simulink model "lead_lag"  (R2015a)
settings: Solver=ode45  StartTime=0.0  StopTime=3999  RelTol=1e-3
undefined symbols (not defined in the file or in its folder): sigbuilder_block
libraries: powerlib_meascontrol x4
settings Model: CovSFcnEnable=off  Creator=MEHRDAD  LastModifiedBy=FaraDars
settings DebuggingCC: SolverPrmCheckMsg=warning

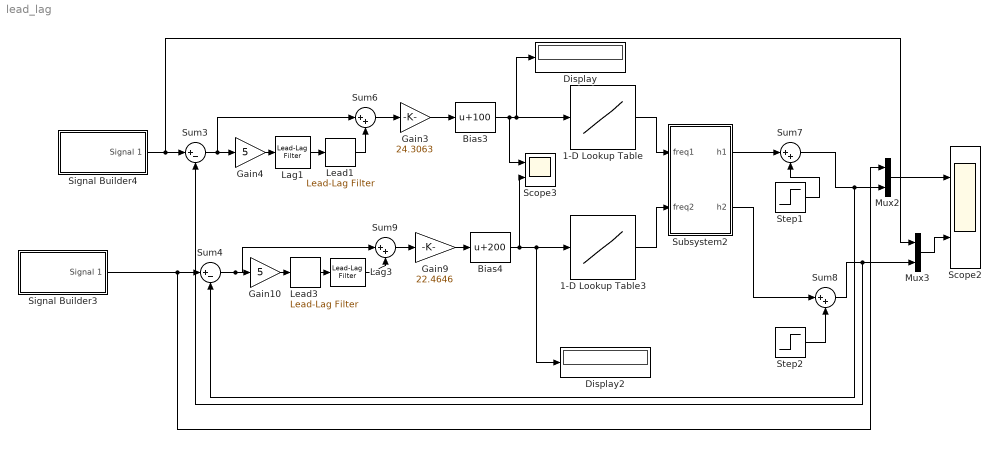
== system lead_lag ==
  1-D Lookup Table : Lookup_n-D  NumberOfTableDimensions=1  BreakpointsForDimension1="[163.87 211.67  227.76 244.4 261.62 274.69 289.41 301.46 318.94 330.75 334.66]"  Table=[21 22 23 24 25 26 27 28 29 30 31]  InternalRulePriority=Speed  RndMeth=Simplest  InputSameDT=on
  1-D Lookup Table3 : Lookup_n-D  NumberOfTableDimensions=1  BreakpointsForDimension1=[ 178.15 234.55 279.97 322.51 357.16 393.93 415.2 473.02 487.03 513.69 555.26 570.95 598.52]  Table=[ 18 19 20 21 22 23 24 25 26 27 28 29 30]  InternalRulePriority=Speed  RndMeth=Simplest  InputSameDT=on
  Bias3 : Bias  Bias=100
  Bias4 : Bias  Bias=200
  Display : Display
  Display2 : Display
  Gain10 : Gain  Gain=5
  Gain3 : Gain  Gain=24.3063
  Gain4 : Gain  Gain=5
  Gain9 : Gain  Gain=22.4646
  Lag1 : powerlib_meascontrol/Filters/Lead-Lag Filter  T1=1/0.001  T2=1/0.0002  Vdc_Init=0  Ts=0
  Lag3 : powerlib_meascontrol/Filters/Lead-Lag Filter  T1=1/0.001  T2=1/0.0002  Vdc_Init=0  Ts=0
  Lead1 : powerlib_meascontrol/Filters/Lead-Lag Filter  T1=13/25  T2=0.052  Vdc_Init=0  Ts=0
  Lead3 : powerlib_meascontrol/Filters/Lead-Lag Filter  T1=13/25  T2=0.052  Vdc_Init=0  Ts=0
  Mux2 : Mux  Inputs=2
  Mux3 : Mux  Inputs=2
  Scope2 : Scope  NumInputPorts=2
      settings: TimeRange=3999  YMin=41.76666666666668~45.27074074074077  YMax=51.36666666666667~45.3240740740741  SaveName=ScopeData5
  Scope3 : Scope  NumInputPorts=2
      settings: YMin=-100~50  YMax=300~400  SaveName=ScopeData6
  Signal Builder3 : Subsystem  Tag=STV Subsys  LoadFcn=sigbuilder_block('load');  StartFcn=sigbuilder_block('start');  StopFcn=sigbuilder_block('stop');  ClipboardFcn=sigbuilder_block('clipboard');  mask(Sigbuilder block){}
      mask help: Simulink:masks:SigbuilderBlock_MD
      mask init:
      | if ~strcmp(get_param(bdroot(gcbh),'SimulationStatus'),'stopped') tuvar = sigbuilder_block('maskInit'); end
      settings: CopyFcn=sigbuilder_block('copy');  DeleteFcn=sigbuilder_block('delete');  ModelCloseFcn=sigbuilder_block('modelClose');  PreSaveFcn=sigbuilder_block('preSave');  PauseFcn=sigbuilder_block('pause');  ContinueFcn=sigbuilder_block('continue');  NameChangeFcn=sigbuilder_block('namechange');  OpenFcn=sigbuilder_block('open',[6 28.5 1011.75 484.5 ]);  CloseFcn=sigbuilder_block('close');
      mask Display: plot(0, 0, 100, 100,[2, 2, 32, 32, 2], [68, 8, 8, 68, 68],[32, 2], [38, 38], [32, 19, 2],[53, 60, 44], [32, 17, 17, 2],[16, 16, 31, 31]);txt = getActiveGroup(gcbh);text(2, 100, txt,'verticalAlignment', 'top');
  Signal Builder4 : Subsystem  Tag=STV Subsys  LoadFcn=sigbuilder_block('load');  StartFcn=sigbuilder_block('start');  StopFcn=sigbuilder_block('stop');  ClipboardFcn=sigbuilder_block('clipboard');  mask(Sigbuilder block){}
      mask help: Simulink:masks:SigbuilderBlock_MD
      mask init:
      | if ~strcmp(get_param(bdroot(gcbh),'SimulationStatus'),'stopped') tuvar = sigbuilder_block('maskInit'); end
      settings: CopyFcn=sigbuilder_block('copy');  DeleteFcn=sigbuilder_block('delete');  ModelCloseFcn=sigbuilder_block('modelClose');  PreSaveFcn=sigbuilder_block('preSave');  PauseFcn=sigbuilder_block('pause');  ContinueFcn=sigbuilder_block('continue');  NameChangeFcn=sigbuilder_block('namechange');  OpenFcn=sigbuilder_block('open',[6 28.5 1011.75 484.5 ]);  CloseFcn=sigbuilder_block('close');
      mask Display: plot(0, 0, 100, 100,[2, 2, 32, 32, 2], [68, 8, 8, 68, 68],[32, 2], [38, 38], [32, 19, 2],[53, 60, 44], [32, 17, 17, 2],[16, 16, 31, 31]);txt = getActiveGroup(gcbh);text(2, 100, txt,'verticalAlignment', 'top');
  Step1 : Step  Time=2000  SampleTime=0
  Step2 : Step  Time=2000  SampleTime=0
  Subsystem2 : Subsystem
  Sum3 : Sum  Inputs=|+-
  Sum4 : Sum  Inputs=|+-
  Sum{6..9} (4 alike) : Sum  Inputs=|++
  wires:
  1-D Lookup Table/1 -> Subsystem2/1(freq1)
  Mux2/1 -> Scope2/1
  Mux3/1 -> Scope2/2
  Bias4/1 -> Scope3/2, 1-D Lookup Table3/1, Display2/1
  Bias3/1 -> 1-D Lookup Table/1, Display/1, Scope3/1
  Signal Builder4/1(Signal 1) -> Mux3/1, Sum3/1
  Signal Builder3/1(Signal 1) -> Mux2/1, Sum4/1
  1-D Lookup Table3/1 -> Subsystem2/2(freq2)
  Sum9/1 -> Gain9/1
  Sum4/1 -> Sum9/1, Gain10/1
  Gain4/1 -> Lag1/1
  Sum6/1 -> Gain3/1
  Sum3/1 -> Sum6/1, Gain4/1
  Gain3/1 -> Bias3/1
  Gain9/1 -> Bias4/1
  Subsystem2/1(h1) -> Sum7/1
  Sum7/1 -> Sum4/2, Mux2/2
  Step1/1 -> Sum7/2
  Subsystem2/2(h2) -> Sum8/1
  Step2/1 -> Sum8/2
  Sum8/1 -> Sum3/2, Mux3/2
  Lag1/1 -> Lead1/1
  Lead1/1 -> Sum6/2
  Lead3/1 -> Lag3/1
  Gain10/1 -> Lead3/1
  Lag3/1 -> Sum9/2

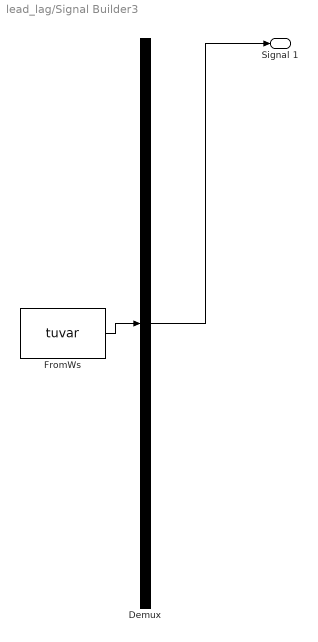
== system lead_lag/Signal Builder3 ==
  Demux : Demux  Tag=STV Demux  Outputs=1
  FromWs : FromWorkspace  Tag=STV FromWs  VariableName=tuvar  SampleTime=0
      SigBuilderData=|
      | common.afterFinalStr = 'Extrapolate'
      | common.sampleTime = 0
      | dataSet.timeRange = [0 3200]
      | dataSet.name = 'Group 1'
      | sbobj.Groups.Name = 'Group 1'
      | sbobj.Groups.Signals.Name = 'Signal 1'
      | sbobj.Groups.Signals.XData = [0 1000 1000 2500 2500 3000 3200]
      | sbobj.Groups.Signals.YData = [42 42 47 47 42 42 42]
      | sbobj.Groups.TimeRange = [0 3200]
  Signal 1 : Outport  Tag=STV Outport
  wires:
  Demux/1 -> Signal 1/1
  FromWs/1 -> Demux/1

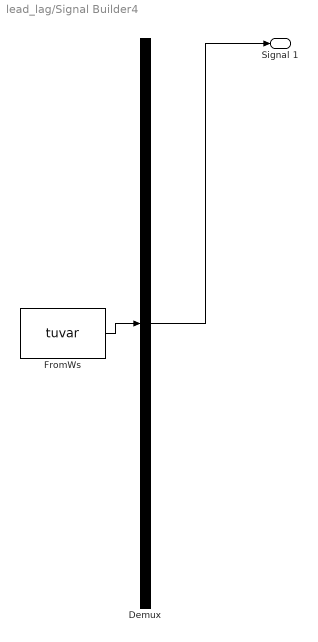
== system lead_lag/Signal Builder4 ==
  Demux : Demux  Tag=STV Demux  Outputs=1
  FromWs : FromWorkspace  Tag=STV FromWs  VariableName=tuvar  SampleTime=0
      SigBuilderData=|
      | common.afterFinalStr = 'Extrapolate'
      | common.sampleTime = 0
      | dataSet.timeRange = [0 3200]
      | dataSet.name = 'Group 1'
      | sbobj.Groups.Name = 'Group 1'
      | sbobj.Groups.Signals.Name = 'Signal 1'
      | sbobj.Groups.Signals.XData = [0 1000 1000 2500 2500 3000 3200]
      | sbobj.Groups.Signals.YData = [40 40 45 45 40 40 40]
      | sbobj.Groups.TimeRange = [0 3200]
  Signal 1 : Outport  Tag=STV Outport
  wires:
  Demux/1 -> Signal 1/1
  FromWs/1 -> Demux/1

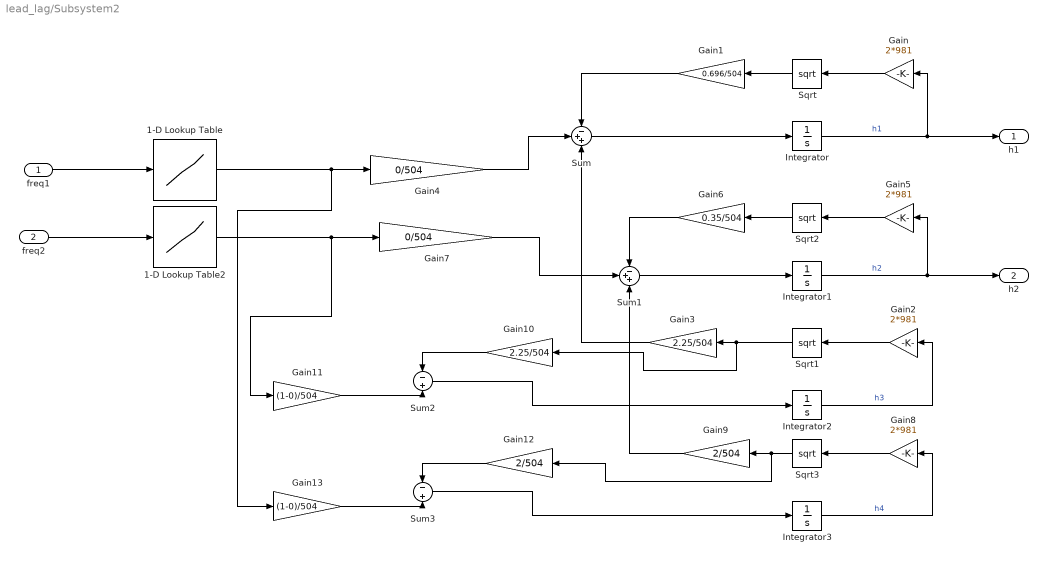
== system lead_lag/Subsystem2 ==
  freq1 : Inport
  freq2 : Inport  Port=2
  1-D Lookup Table : Lookup_n-D  NumberOfTableDimensions=1  BreakpointsForDimension1=[21 22 23 24 25 26 27 28 29 30 31]  Table="[163.87 211.67  227.76 244.4 261.62 274.69 289.41 301.46 318.94 330.75 334.66]"  InternalRulePriority=Speed  RndMeth=Simplest  InputSameDT=on
  1-D Lookup Table2 : Lookup_n-D  NumberOfTableDimensions=1  BreakpointsForDimension1=[18 19 20 21 22 23 24 25 26 27 28 29 30]  Table=[ 178.15 234.55 279.97 322.51 357.16 393.93 415.2 473.02 487.03 513.69 555.26 570.95 598.52]  InternalRulePriority=Speed  RndMeth=Simplest  InputSameDT=on
  Gain{,2,5,8} (4 alike) : Gain  Gain=2*981
  Gain1 : Gain  Gain=0.696/504
  Gain10 : Gain  Gain=2.25/504
  Gain11 : Gain  Gain=(1-0)/504
  Gain12 : Gain  Gain=2/504
  Gain13 : Gain  Gain=(1-0)/504
  Gain3 : Gain  Gain=2.25/504
  Gain4 : Gain  Gain=0/504
  Gain6 : Gain  Gain=0.35/504
  Gain7 : Gain  Gain=0/504
  Gain9 : Gain  Gain=2/504
  Integrator{,1..3} (4 alike) : Integrator  LimitOutput=on  LowerSaturationLimit=0
  Sqrt{,1..3} (4 alike) : Sqrt  SaturateOnIntegerOverflow=on
  Sum : Sum  Inputs=-++
  Sum1 : Sum  Inputs=-++
  Sum2 : Sum  Inputs=-+
  Sum3 : Sum  Inputs=-+
  h1 : Outport
  h2 : Outport  Port=2
  wires:
  Sqrt3/1 -> Gain12/1, Gain9/1
  Integrator3/1 -> Gain8/1  "h4"
  Gain9/1 -> Sum1/3
  Gain8/1 -> Sqrt3/1
  Sum2/1 -> Integrator2/1
  Integrator/1 -> Gain/1, h1/1  "h1"
  Integrator2/1 -> Gain2/1  "h3"
  Gain3/1 -> Sum/3
  Gain2/1 -> Sqrt1/1
  Gain/1 -> Sqrt/1
  Sqrt/1 -> Gain1/1
  Sqrt1/1 -> Gain10/1, Gain3/1
  Gain1/1 -> Sum/1
  Integrator1/1 -> h2/1, Gain5/1  "h2"
  Sum/1 -> Integrator/1
  Gain4/1 -> Sum/2
  Sum3/1 -> Integrator3/1
  Gain7/1 -> Sum1/2
  Gain5/1 -> Sqrt2/1
  Sqrt2/1 -> Gain6/1
  Sum1/1 -> Integrator1/1
  Gain10/1 -> Sum2/1
  Gain11/1 -> Sum2/2
  Gain13/1 -> Sum3/2
  Gain6/1 -> Sum1/1
  Gain12/1 -> Sum3/1
  freq1/1 -> 1-D Lookup Table/1
  freq2/1 -> 1-D Lookup Table2/1
  1-D Lookup Table/1 -> Gain13/1, Gain4/1
  1-D Lookup Table2/1 -> Gain11/1, Gain7/1
